simulink model "Laba1"  (R2017b)
settings: Solver=ode45  StartTime=0.0  StopTime=0.01  MaxStep=0.01  RelTol=1e-3
values from neighbouring files (symbols this model uses):
  C = 10e-6    (= 1e-05)    [Laba1_data.m]
  Em = 36    [Laba1_data.m]
  f = 50    [Laba1_data.m]
  L = 3e-3    (= 0.003)    [Laba1_data.m]
  R1 = 15    [Laba1_data.m]
  R2 = 25    [Laba1_data.m]
libraries: fl_lib x8, nesl_utility x4
settings Model: Creator=Aleksandr  LastModifiedBy=Aleksandr

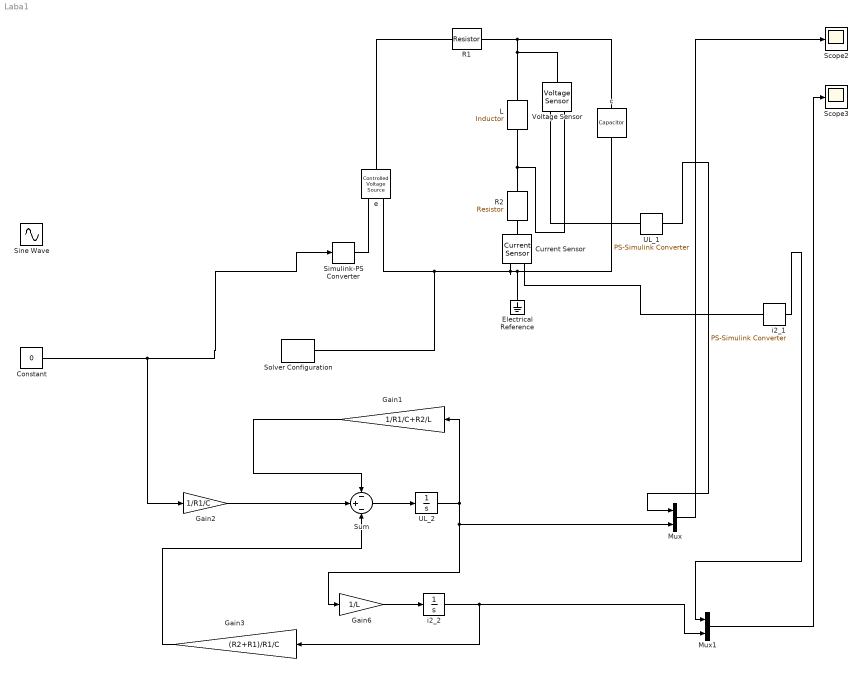
== system Laba1 ==
  Constant : Constant  Value=0
  Current Sensor : fl_lib/Electrical/Electrical Sensors/Current Sensor
  Electrical Reference : fl_lib/Electrical/Electrical Elements/Electrical Reference
  Gain1 : Gain  Gain=1/R1/C+R2/L
  Gain2 : Gain  Gain=1/R1/C
  Gain3 : Gain  Gain=(R2+R1)/R1/C
  Gain6 : Gain  Gain=1/L
  L : fl_lib/Electrical/Electrical Elements/Inductor  l=L H  r=0 Ohm  g=1e-9 1/Ohm  i_specify=off  i_priority=High  i=2 A  i_nominal_specify=off  i_nominal_unit=A  i_nominal_value=1  v_specify=off  v_priority=Low  v=40 V  v_nominal_specify=off  v_nominal_unit=V  v_nominal_value=1  i_L_specify=on  i_L_priority=High  i_L=2 A  i_L_nominal_specify=off  i_L_nominal_unit=A  i_L_nominal_value=1
  Mux : Mux  Inputs=2
  Mux1 : Mux  Inputs=2
  R1 : fl_lib/Electrical/Electrical Elements/Resistor  R=R1 Ohm  i_specify=off  i_priority=None  i=0 A  i_nominal_specify=off  i_nominal_unit=A  i_nominal_value=1  v_specify=off  v_priority=High  v=-20 V  v_nominal_specify=off  v_nominal_unit=V  v_nominal_value=1
  R2 : fl_lib/Electrical/Electrical Elements/Resistor  R=R2 Ohm  i_specify=off  i_priority=High  i=-2 A  i_nominal_specify=off  i_nominal_unit=A  i_nominal_value=1  v_specify=off  v_priority=High  v=-40 V  v_nominal_specify=off  v_nominal_unit=V  v_nominal_value=1
  Scope2 : Scope
  Scope3 : Scope
  Simulink-PS Converter : nesl_utility/Simulink-PS Converter  PhysicalDomain=network_engine_domain  SubClassName=ps_input  LeftPortType=input  RightPortType=output  PseudoPeriodic=off  Frequencies=[]  NoiseDistribution=none  NoiseParameters=[]  Unit=V  AffineConversion=off  FilteringAndDerivatives=provide  SimscapeFilterOrder=1  InputFilterTimeConstant=0.001  UdotUserProvided=0
  Sine Wave : Sin  Amplitude=Em  Frequency=2*pi*f  SampleTime=0
  Solver Configuration : nesl_utility/Solver Configuration  PhysicalDomain=network_engine_domain  SubClassName=solver  LeftPortType=input  RightPortType=generic  Accelerate=off  Tones=[]  Harmonics=[]  SimulateNoise=off  Profile=off  UseLocalSampling=off  EnableSwitchedLinearOptims=on  FrequencyDomain=off  UseCCode=off  RelTol=0.001  AbsTol=1e-06  MinStep=1e-09  ToWorkspace=off  RevertToSquareIcSolve=off  NumHomotopyIterations=100  PhasorMode=off  PhasorModeNumHarmonics=1  DoDC=off  ResidualTolerance=1e-09  UseLocalSolver=off  LocalSolverChoice=NE_BACKWARD_EULER_ADVANCER  LocalSolverSampleTime=0.001  DoFixedCost=off  MaxNonlinIter=3  MaxModeIter=2  LinearAlgebra=Sparse  DelaysMemoryBudget=1024  AutomaticFiltering=on  FilteringTimeConstant=0.001
  Sum : Sum  Inputs=-+-
  UL_1 : nesl_utility/PS-Simulink Converter  PhysicalDomain=network_engine_domain  SubClassName=ps_output  LeftPortType=input  RightPortType=output  PseudoPeriodic=off  Frequencies=[]  Unit=1  AffineConversion=off
  UL_2 : Integrator  InitialCondition=-40
  Voltage Sensor : fl_lib/Electrical/Electrical Sensors/Voltage Sensor
  c : fl_lib/Electrical/Electrical Elements/Capacitor  c=C F  r=1e-6 Ohm  g=0 1/Ohm  i_specify=off  i_priority=None  i=0 A  i_nominal_specify=off  i_nominal_unit=A  i_nominal_value=1  v_specify=off  v_priority=High  v=5 V  v_nominal_specify=off  v_nominal_unit=V  v_nominal_value=1  vc_specify=on  vc_priority=High  vc=10 V  vc_nominal_specify=off  vc_nominal_unit=V  vc_nominal_value=1
  e : fl_lib/Electrical/Electrical Sources/Controlled Voltage Source
  i2_1 : nesl_utility/PS-Simulink Converter  PhysicalDomain=network_engine_domain  SubClassName=ps_output  LeftPortType=input  RightPortType=output  PseudoPeriodic=off  Frequencies=[]  Unit=1  AffineConversion=off
  i2_2 : Integrator  InitialCondition=2
  wires:
  UL_1/1 -> Mux/1
  i2_1/1 -> Mux1/1
  Constant/1 -> Gain2/1, Simulink-PS Converter/1
  Sum/1 -> UL_2/1
  UL_2/1 -> Gain1/1, Gain6/1, Mux/2
  Mux/1 -> Scope2/1
  Mux1/1 -> Scope3/1
  i2_2/1 -> Gain3/1, Mux1/2
  Gain6/1 -> i2_2/1
  Gain1/1 -> Sum/1
  Gain2/1 -> Sum/2
  Gain3/1 -> Sum/3
  connections:
  R1/LConn1 -- e/LConn1
  L/LConn1 -- Voltage Sensor/LConn1 -- c/LConn1 -- R1/RConn1
  L/RConn1 -- Voltage Sensor/RConn2 -- R2/LConn1
  e/RConn2 -- Solver Configuration/RConn1 -- Current Sensor/RConn2 -- c/RConn1 -- Electrical Reference/LConn1
  Simulink-PS Converter/RConn1 -- e/RConn1
  Voltage Sensor/RConn1 -- UL_1/LConn1
  Current Sensor/LConn1 -- R2/RConn1
  Current Sensor/RConn1 -- i2_1/LConn1
